simulink model "iiwa_IK_ROS"  (R2016b)
settings: Solver=FixedStepAuto  StartTime=0.0  StopTime=inf  FixedStep=0.05  RelTol=1e-3
model workspace (MAT data in the model file):
  SL_ROS_VariableLengthArrays_MaxSizes : struct (value not decoded)
libraries: robotlib x5
(part 3 of 3)

== matlab function iiwa_IK_ROS/error_calc ==
  data: tf_in_msg input Bus: SL_Bus_iiwa_IK_ROS_tf2_msgs_TFMessage; E output double; en1 output; en2 output; tf_n output; x output; y output; z output
% Based on transformation between /iiwa_base_link and /target_frame from tf
% as on error IK problem is solved and corresponding joint angles 
% changes is sent to arm_state topic

function [E,en1,en2,tf_n,x,y,z]  = fcn(tf_in_msg)

en1 = 0;
en2 = 0;
persistent E1;
persistent E2;
persistent E3;
persistent E4;
persistent E5;
persistent E6;
if isempty(E1)
    E1 = double(0.0);
end
if isempty(E2)
    E2 = double(0.0);
end
if isempty(E3)
    E3 = double(0.0);
end
if isempty(E4)
    E4 = double(0.0);
end
if isempty(E5)
    E5 = double(0.0);
end
if isempty(E6)
    E6 = double(0.0);
end


%sec = 0.0;
tf_n = tf_in_msg.Transforms_SL_Info.CurrentLength;
%if (tf_nums > 1)
%    sec = tf_msg_in.Transforms(1).Header.Stamp.Sec;
%end

%%%%%%%%%%%%%%%%%%%%%%%%%%%%%%%%%%%%%%%%%%%%%%%%
par = 'iiwa_base_link';
ch1 = 'error';
x=0;
y=0;
z=0;
% referenceString = 'right-e0';
% maxStrings = length(msg.Name);
% numStrings = msg.Name_SL_Info.CurrentLength;
% 
% foundIndex = -1;
% for i=1:numStrings
%     if compareString(msg, i, referenceString)
%         foundIndex = double(i);
%         break;
%     end
% end
%%%%%%%%%%%%%%%%%%%%%%%%%%%%%%%%%%%%%%%%%%%%%%%%%%%%%

%for i=1:tf_n
if (tf_n==1)
    i=1;
    child_fr = tf_in_msg.Transforms(i).ChildFrameId;
    parent_fr = tf_in_msg.Transforms(i).Header.FrameId;
    if (strncmp(char(parent_fr), par, length(par)))
       en1 = 1;
       if (strncmp(char(child_fr), ch1, length(ch1)))
           en2 = 1;
           x = tf_in_msg.Transforms(i).Transform.Translation.X;
           y = tf_in_msg.Transforms(i).Transform.Translation.Y;
           z = tf_in_msg.Transforms(i).Transform.Translation.Z;
           E1 = tf_in_msg.Transforms(i).Transform.Translation.X;
           E2 = tf_in_msg.Transforms(i).Transform.Translation.Y;
           E3 = tf_in_msg.Transforms(i).Transform.Translation.Z;
           eul = quat2eul([tf_in_msg.Transforms(i).Transform.Rotation.W,...
                                tf_in_msg.Transforms(i).Transform.Rotation.X,...
                                tf_in_msg.Transforms(i).Transform.Rotation.Y,...
                                tf_in_msg.Transforms(i).Transform.Rotation.Z,]);
           E4 = eul(3);
           E5 = eul(2);
           E6 = eul(1); 
       end
    end

    %en = 2;
    %str = double(parent_fr);
%     str_length = length(str);
%     control_js_msg.Name(idx).Data(1:str_length) = uint8(str);
%     control_js_msg.Name(idx).Data_SL_Info.CurrentLength = uint32(str_length);
end

E = double([E1;E2;E3;E4;E5;E6]);
%E = [0;0;0;0;0;0];

end

%%------------
% function isMatch = compareString(msg, index, strToCheck)
% 
% % Check for an exact match to strToCheck 
% isMatch = strncmp(char(msg.Name(index).Data), strToCheck, length(strToCheck));
% 
% % Alternative manipulation:
% %  Check only through msg.Data_SL_Info.CurrentLength. This allows substring
% %  matches (i.e., if the received string is shorter than strToCheck)
% %
% %  isMatch = strncmp(char(msg.Data), strToCheck, msg.Data_SL_Info.CurrentLength);
% end


% function [control_js_msg, H] = fcn(blank_js_msg, ctrl)
% 
% persistent seq;
% if isempty(seq)
%     seq = 0;
% end
% 
% str_array_of_jnames = {'iiwa_j1', 'iiwa_j2', 'iiwa_j3', 'iiwa_j4', 'iiwa_j5', 'iiwa_j6', 'iiwa_j7'};
% control_js_msg = blank_js_msg;
% 
% th_num = length(str_array_of_jnames);
% control_js_msg.Name_SL_Info.CurrentLength = uint32(th_num);
% 
% %sec = 0.0;
% %tf_nums = tf_msg_in.Transforms_SL_Info.CurrentLength;
% %if (tf_nums > 1)
% %    sec = tf_msg_in.Transforms(1).Header.Stamp.Sec;
% %end
% 
% for idx=1:th_num
%     str = str_array_of_jnames{idx};
%     str_length = length(str);
%     control_js_msg.Name(idx).Data(1:str_length) = uint8(str);
%     control_js_msg.Name(idx).Data_SL_Info.CurrentLength = uint32(str_length);
% end
%                                                                                                                                                                                                                                                                                                                                                                                                                                                                         0,                                                                                                                                                                                                                                                                                                                                                                                                                                                                  0,                                                                                                                                                                                                                                                                              0,                                                                                                                                                                                                                                                                                                                                                                                                           1];  
%      
% control_js_msg.Header.Seq = uint32(seq);
% seq = seq + 1;
% end
